simulink model "aerosonde_demo6"  (Simulink 4.0)
settings: Solver=ode4  StartTime=0.0  StopTime=300  FixedStep=0.05  RelTol=1e-3
libraries: simulink_extras x5, aerosimlib x2
settings Model: LastModifiedBy=mariusn  SaveTime=off  SaveOutput=off  LimitDataPoints=off  UnconnectedInputMsg=none  UnconnectedOutputMsg=none  UnconnectedLineMsg=none  BlockReductionOpt=off

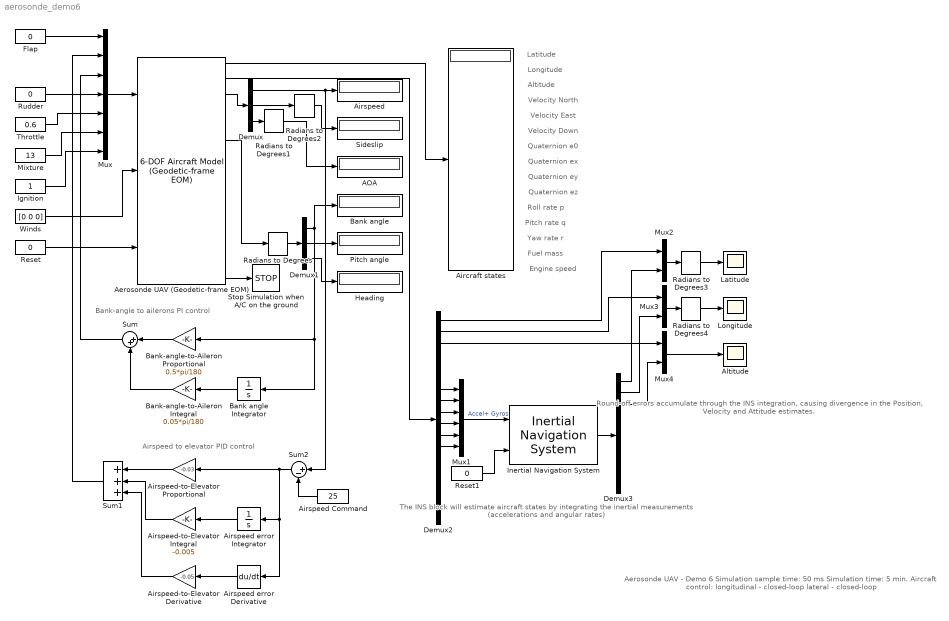
== system aerosonde_demo6 ==
  note: Velocity North
  note: Velocity East
  note: Velocity Down
  note: Roll rate p
  note: Pitch rate q
  note: Yaw rate r
  note: Quaternion e0
  note: Quaternion ex
  note: Quaternion ey
  note: Quaternion ez
  note: Latitude
  note: Longitude
  note: Altitude
  note: Fuel mass
  note: Engine speed
  note: Aerosonde UAV - Demo 6
      | Simulation sample time: 50 ms
      | Simulation time: 5 min.
      | Aircraft control: longitudinal - closed-loop
      |                  lateral - closed-loop
  note: Bank-angle to ailerons PI control
  note: Airspeed to elevator PID control
  note: Round-off errors accumulate through the INS integration,
      | causing divergence in the Position, Velocity and Attitude
      | estimates.
  note: The INS block will estimate aircraft states by
      | integrating the inertial measurements
      | (accelerations and angular rates)
  AOA : Display
      settings: Format=short
  Aerosonde UAV (Geodetic-frame EOM) : aerosimlib/Complete Aircraft/6-DOF Aircraft Model (Geodetic-frame EOM)  aircraftcfg='aerosondecfg.mat'  PositionIni=[45*pi/180 -122*pi/180 1000]'  VelocitiesIni=[23 0 0]'  QuaternionsIni=[1 0 0 0]'  RatesIni=[0 0 0]'  FuelIni=2  OmegaIni=5000*pi/30  GndAlt=20  wmmfile='C:\Program Files\AeroSim\wmm.cof'  dmy=[09 01 2002]  tsamp=0.05
  Aircraft states : Display
      settings: Format=short
  Airspeed : Display
      settings: Format=short
  Airspeed Command : Constant  Orientation=left  Value=25
  Airspeed error Derivative : Derivative  Orientation=left
  Airspeed error Integrator : Integrator  Orientation=left  ExternalReset=none  InitialConditionSource=internal  InitialCondition=0  LimitOutput=off  UpperSaturationLimit=inf  LowerSaturationLimit=-inf  ShowSaturationPort=off  ShowStatePort=off  AbsoluteTolerance=auto
  Airspeed-to-Elevator Derivative : Gain  Orientation=left  Gain=-0.05  Multiplication=Element-wise(K.*u)  SaturateOnIntegerOverflow=on
  Airspeed-to-Elevator Integral : Gain  Orientation=left  Gain=-0.005  Multiplication=Element-wise(K.*u)  SaturateOnIntegerOverflow=on
  Airspeed-to-Elevator Proportional : Gain  Orientation=left  Gain=-0.03  Multiplication=Element-wise(K.*u)  SaturateOnIntegerOverflow=on
  Altitude : Scope
      settings: TimeRange=300  YMin=900  YMax=1000  SaveToWorkspace=off  SaveName=ScopeData2  MaxDataPoints=5000
  Bank angle : Display
      settings: Format=short
  Bank angle Integrator : Integrator  Orientation=left  ExternalReset=none  InitialConditionSource=internal  InitialCondition=0  LimitOutput=off  UpperSaturationLimit=inf  LowerSaturationLimit=-inf  ShowSaturationPort=off  ShowStatePort=off  AbsoluteTolerance=auto
  Bank-angle-to-Aileron Integral : Gain  Orientation=left  Gain=0.05*pi/180  Multiplication=Element-wise(K.*u)  SaturateOnIntegerOverflow=on
  Bank-angle-to-Aileron Proportional : Gain  Orientation=left  Gain=0.5*pi/180  Multiplication=Element-wise(K.*u)  SaturateOnIntegerOverflow=on
  Demux : Demux  Outputs=3  BusSelectionMode=off
  Demux1 : Demux  Outputs=3  BusSelectionMode=off
  Demux2 : Demux  Outputs=18  BusSelectionMode=off
  Demux3 : Demux  Outputs=10  BusSelectionMode=off
  Flap : Constant  Value=0
  Heading : Display
      settings: Format=short
  Ignition : Constant  Value=1
  Inertial Navigation System : aerosimlib/Complete Aircraft/Inertial Navigation System  PositionIni=[45*pi/180 -122*pi/180 1000]'  VelocitiesIni=[23 0 0]'  QuaternionsIni=[1 0 0 0]'  tsamp=0.05
  Latitude : Scope
      settings: TimeRange=300  YMin=45  YMax=45.08  SaveToWorkspace=off  SaveName=ScopeData  MaxDataPoints=5000
  Longitude : Scope
      settings: TimeRange=300  YMin=-122.01  YMax=-121.996  SaveToWorkspace=off  MaxDataPoints=5000
  Mixture : Constant  Value=13
  Mux : Mux  Inputs=7
  Mux1 : Mux  Inputs=6
  Mux2 : Mux  Inputs=2
  Mux3 : Mux  Inputs=2
  Mux4 : Mux  Inputs=2
  Pitch angle : Display
      settings: Format=short
  Radians to Degrees{,1..4} (5 alike) : simulink_extras/Transformations/Radians to Degrees
  Reset : Constant  Value=0
  Reset1 : Constant  Value=0
  Rudder : Constant  Value=0
  Sideslip : Display
      settings: Format=short
  Stop Simulation when A/C on the ground : Stop
  Sum : Sum  Orientation=left  Inputs=|++  SaturateOnIntegerOverflow=on
  Sum1 : Sum  Orientation=left  Inputs=+++  SaturateOnIntegerOverflow=on
  Sum2 : Sum  Orientation=left  Inputs=|+-  SaturateOnIntegerOverflow=on
  Throttle : Constant  Value=0.6
  Winds : Constant  Value=[0 0 0]
  wires:
  Reset/1 -> Aerosonde UAV (Geodetic-frame EOM)/3
  Winds/1 -> Aerosonde UAV (Geodetic-frame EOM)/2
  Aerosonde UAV (Geodetic-frame EOM)/1 -> Aircraft states/1
  Aerosonde UAV (Geodetic-frame EOM)/6 -> Radians to Degrees/1
  Aerosonde UAV (Geodetic-frame EOM)/3 -> Demux/1
  Demux/3 -> Radians to Degrees1/1
  Demux/2 -> Radians to Degrees2/1
  Demux/1 -> Airspeed/1, Sum2/1
  Radians to Degrees2/1 -> Sideslip/1
  Radians to Degrees1/1 -> AOA/1
  Aerosonde UAV (Geodetic-frame EOM)/15 -> Stop Simulation when A/C on the ground/1
  Radians to Degrees/1 -> Demux1/1
  Demux1/2 -> Pitch angle/1
  Demux1/3 -> Heading/1
  Demux1/1 -> Bank angle/1, Bank-angle-to-Aileron Proportional/1, Bank angle Integrator/1
  Flap/1 -> Mux/1
  Rudder/1 -> Mux/4
  Throttle/1 -> Mux/5
  Mixture/1 -> Mux/6
  Ignition/1 -> Mux/7
  Mux/1 -> Aerosonde UAV (Geodetic-frame EOM)/1
  Bank-angle-to-Aileron Proportional/1 -> Sum/1
  Bank angle Integrator/1 -> Bank-angle-to-Aileron Integral/1
  Bank-angle-to-Aileron Integral/1 -> Sum/2
  Sum/1 -> Mux/3
  Airspeed error Derivative/1 -> Airspeed-to-Elevator Derivative/1
  Airspeed error Integrator/1 -> Airspeed-to-Elevator Integral/1
  Airspeed-to-Elevator Proportional/1 -> Sum1/1
  Airspeed-to-Elevator Integral/1 -> Sum1/2
  Airspeed-to-Elevator Derivative/1 -> Sum1/3
  Sum1/1 -> Mux/2
  Sum2/1 -> Airspeed-to-Elevator Proportional/1, Airspeed error Integrator/1, Airspeed error Derivative/1
  Airspeed Command/1 -> Sum2/2
  Aerosonde UAV (Geodetic-frame EOM)/2 -> Demux2/1
  Demux2/7 -> Mux1/1
  Demux2/8 -> Mux1/2
  Demux2/9 -> Mux1/3
  Demux2/10 -> Mux1/4
  Demux2/11 -> Mux1/5
  Demux2/12 -> Mux1/6
  Mux1/1 -> Inertial Navigation System/1  "Accel+ Gyros"
  Reset1/1 -> Inertial Navigation System/2
  Inertial Navigation System/1 -> Demux3/1
  Mux2/1 -> Radians to Degrees3/1
  Mux3/1 -> Radians to Degrees4/1
  Mux4/1 -> Altitude/1
  Radians to Degrees3/1 -> Latitude/1
  Radians to Degrees4/1 -> Longitude/1
  Demux2/1 -> Mux2/1
  Demux2/2 -> Mux3/1
  Demux2/3 -> Mux4/1
  Demux3/1 -> Mux2/2
  Demux3/2 -> Mux3/2
  Demux3/3 -> Mux4/2
